simulink model "OPC_AUTOMATIZACIO_PROCESOS"  (R2014b)
settings: Solver=ode45  StartTime=0.0  StopTime=inf  RelTol=1e-3
libraries: opclib x6
settings Model: Creator=user  LastModifiedBy=CONTROL02

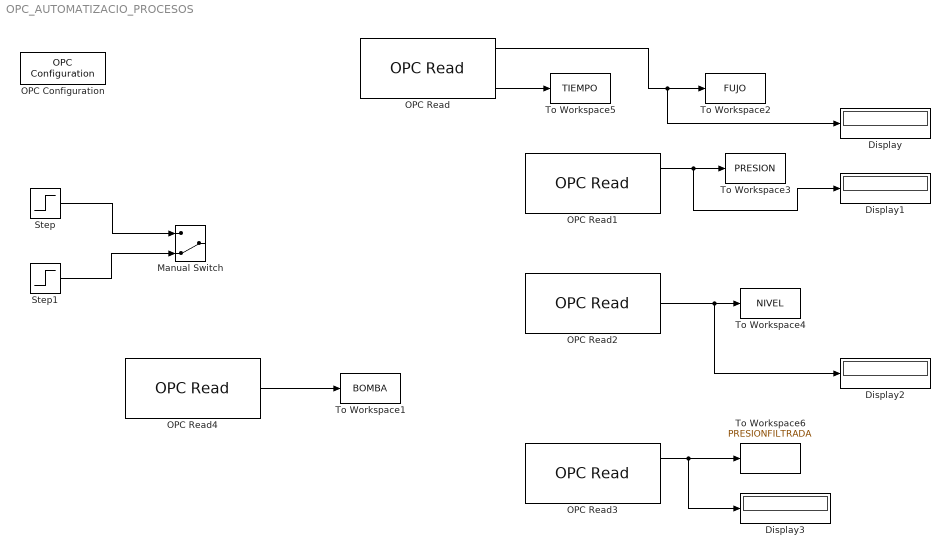
== system OPC_AUTOMATIZACIO_PROCESOS ==
  Display{,1..3} (4 alike) : Display
  Manual Switch : ManualSwitch  CurrentSetting=0
  OPC Configuration : opclib/OPC Configuration  opcServers=localhost/Kepware.KEPServerEX.V6/10  errMissingItems=Error  errReadWrite=Warn  errShutdown=Error  errRTViolation=Warn  rtEnable=on  speedup=1  showLatency=off  beingUsed=on
  OPC Read : opclib/OPC Read  serverHost=localhost  serverID=Kepware.KEPServerEX.V6  itemIDs=1500.Device1.FLUJO  readMode=Synchronous (cache)  dataType=double  updateRate=0  showQual=on  showTS=on  tsMode=Seconds since start
  OPC Read1 : opclib/OPC Read  serverHost=localhost  serverID=Kepware.KEPServerEX.V6  itemIDs=1500.Device1.PRESION  readMode=Synchronous (cache)  dataType=double  updateRate=0  showQual=off  showTS=on  tsMode=Seconds since start
  OPC Read2 : opclib/OPC Read  serverHost=localhost  serverID=Kepware.KEPServerEX.V6  itemIDs=1500.Device1.NIVEL  readMode=Synchronous (cache)  dataType=double  updateRate=0  showQual=off  showTS=off  tsMode=Seconds since start
  OPC Read3 : opclib/OPC Read  serverHost=localhost  serverID=Kepware.KEPServerEX.V6  itemIDs=1500.Device1.FILTROPRESION  readMode=Synchronous (cache)  dataType=double  updateRate=0  showQual=off  showTS=on  tsMode=Seconds since start
  OPC Read4 : opclib/OPC Read  serverHost=localhost  serverID=Kepware.KEPServerEX.V6  itemIDs=1500.Device1.BOMBA  readMode=Synchronous (cache)  dataType=double  updateRate=0  showQual=off  showTS=off  tsMode=Seconds since start
  Step : Step  Time=0  After=27000  SampleTime=0
  Step1 : Step  Time=0  After=7000  SampleTime=0
  To Workspace1 : ToWorkspace  VariableName=BOMBA  SampleTime=-1
  To Workspace2 : ToWorkspace  VariableName=FUJO  SampleTime=-1
  To Workspace3 : ToWorkspace  VariableName=PRESION  SampleTime=-1
  To Workspace4 : ToWorkspace  VariableName=NIVEL  SampleTime=-1
  To Workspace5 : ToWorkspace  VariableName=TIEMPO  SampleTime=-1
  To Workspace6 : ToWorkspace  VariableName=PRESIONFILTRADA  SampleTime=-1
  wires:
  Step/1 -> Manual Switch/1
  Step1/1 -> Manual Switch/2
  OPC Read/1 -> Display/1, To Workspace2/1
  OPC Read1/1 -> Display1/1, To Workspace3/1
  OPC Read2/1 -> Display2/1, To Workspace4/1
  OPC Read/3 -> To Workspace5/1
  OPC Read3/1 -> Display3/1, To Workspace6/1
  OPC Read4/1 -> To Workspace1/1
